simulink model "pvmodelling"  (R2022a)
settings: Solver=FixedStepAuto  StartTime=0.0  StopTime=0.33  FixedStep=0.01  MaxStep=1e-5  MinStep=1e-6  RelTol=1e-6  AbsTol=1e-6  EnableMultiTasking=on
values from neighbouring files (symbols this model uses):
  a1 = x(i,4)    [comp3.m]
  a2 = x(i,5)    [comp3.m]
  I01 = x(i,2)    [comp3.m]    (also in modified_two_diode_model2.m = (B/rp)*(rp+rs))
  I02 = x(i,3)    [comp3.m]    (also in modified_two_diode_model2.m = (E/rp)*(rp+rs))
  Iph = x(i,1)    [comp3.m]    (also in modified_two_diode_model2.m = (A/rp)*(rp+rs))
  Rp = x(i,7)    [comp3.m]
  Rs = x(i,6)    [comp3.m]
  Vt = (K11*(T)*Ns)/Q    (= 0.0828298974046)    [input2.m]
undefined symbols (not defined in the file or in its folder): sigbuilder_block
settings Model: Creator=SREEKANTHA  LastModifiedBy=abdul
settings SolverCC: AutoScaleAbsTol=off  InitialStep=1e-6  AlgebraicLoopSolver=TrustRegion
settings DataIOCC: ReturnWorkspaceOutputs=off
settings OptimizationCC: LifeSpan=inf
settings DebuggingCC: UnconnectedInputMsg=warning  UnconnectedOutputMsg=warning  UnconnectedLineMsg=warning  SFUnexpectedBacktrackingDiag=warning  SFNoUnconditionalDefaultTransitionDiag=warning  SFMachineParentedDataDiag=warning  ArithmeticOperatorsInVariantConditions=warning
settings SFSimCC: SimUseLocalCustomCode=off  CustomCodeUndefinedFunction=UseInterfaceOnly
settings RTWCC: RTWUseLocalCustomCode=off
settings CodeAppCC: StateflowObjectComments=on
settings GRTTargetCC: TargetLangStandard=C89/C90 (ANSI)
settings ConfigComp: CovMetricSettings=dw  CovSaveCumulativeToWorkspaceVar=on  CovSaveSingleToWorkspaceVar=on  CovExternalEMLEnable=off
settings SimscapeCC: SimscapeNormalizeSystem=off

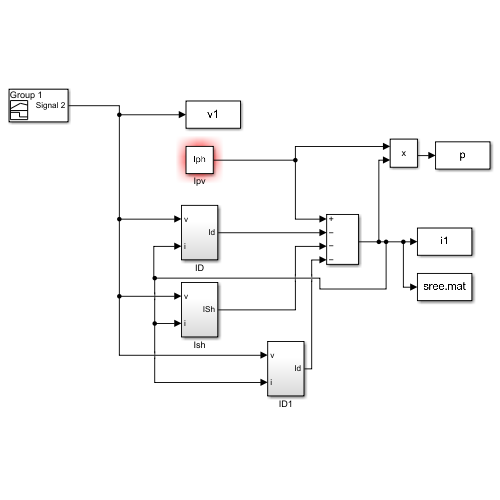
[thumbnail: Simulink's stored preview of the top-level diagram]
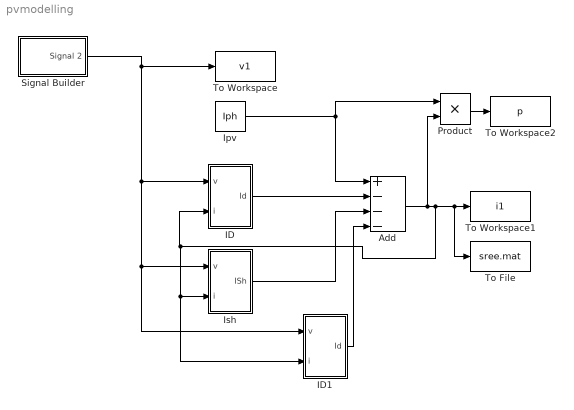
== system pvmodelling ==
  Add : Sum  Inputs=+---
  ID : Subsystem
  ID1 : Subsystem
  Ipv : Constant  Value=Iph
  Ish : Subsystem
  Product : Product
  Signal Builder : Subsystem  Tag=STV Subsys  LoadFcn=sigbuilder_block('load');  StartFcn=sigbuilder_block('start');  StopFcn=sigbuilder_block('stop');  ClipboardFcn=sigbuilder_block('clipboard');  mask(Sigbuilder block){tuvar=[0:10]}
      mask help: Simulink:masks:SigbuilderBlock_MD
      mask init:
      | if ~strcmp(get_param(bdroot(gcbh),'SimulationStatus'),'stopped') tuvar = sigbuilder_block('maskInit'); end
      settings: CopyFcn=sigbuilder_block('copy');  DeleteFcn=sigbuilder_block('delete');  ModelCloseFcn=sigbuilder_block('modelClose');  PreSaveFcn=sigbuilder_block('preSave');  PauseFcn=sigbuilder_block('pause');  ContinueFcn=sigbuilder_block('continue');  NameChangeFcn=sigbuilder_block('namechange');  OpenFcn=sigbuilder_block('open',[0 36 1152 555.6 ]);  CloseFcn=sigbuilder_block('close');
      mask Display: plot(0, 0, 100, 100,[2, 2, 32, 32, 2], [68, 8, 8, 68, 68],[32, 2], [38, 38], [32, 19, 2],[53, 60, 44], [32, 17, 17, 2],[16, 16, 31, 31]);txt = getActiveGroup(gcbh);text(2, 100, txt,'verticalAlignment', 'top');
  To File : ToFile  Filename=sree.mat  MatrixName=ii
  To Workspace : ToWorkspace  VariableName=v1  SampleTime=-1
  To Workspace1 : ToWorkspace  VariableName=i1  SampleTime=-1
  To Workspace2 : ToWorkspace  VariableName=p  SampleTime=-1
  wires:
  Ipv/1 -> Product/1, Add/1
  ID/1(Id) -> Add/2
  Ish/1(ISh) -> Add/3
  Add/1 -> Product/2, To Workspace1/1, To File/1, ID1/2(i), Ish/2(i), ID/2(i)
  Product/1 -> To Workspace2/1
  ID1/1(Id) -> Add/4
  Signal Builder/1(Signal 2) -> ID1/1(v), Ish/1(v), ID/1(v), To Workspace/1

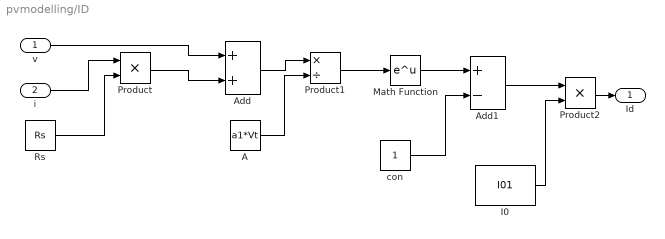
== system pvmodelling/ID ==
  v : Inport
  i : Inport  Port=2
  A : Constant  Value=a1*Vt
  Add : Sum
  Add1 : Sum  Inputs=+-
  I0 : Constant  Value=I01
  Math Function : Math  SignedPower=on
  Product : Product
  Product1 : Product  Inputs=*/
  Product2 : Product
  Rs : Constant  Value=Rs
  con : Constant
  Id : Outport
  wires:
  con/1 -> Add1/2
  Add1/1 -> Product2/1
  Product1/1 -> Math Function/1
  Product/1 -> Add/2
  I0/1 -> Product2/2
  Math Function/1 -> Add1/1
  Product2/1 -> Id/1
  v/1 -> Add/1
  Rs/1 -> Product/2
  A/1 -> Product1/2
  Add/1 -> Product1/1
  i/1 -> Product/1

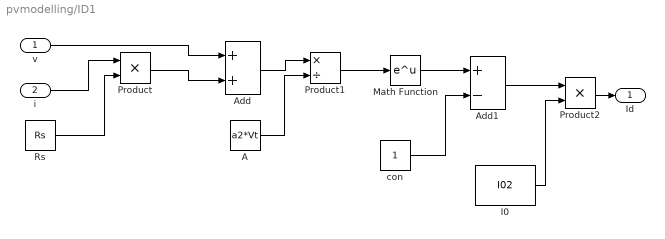
== system pvmodelling/ID1 ==
  v : Inport
  i : Inport  Port=2
  A : Constant  Value=a2*Vt
  Add : Sum
  Add1 : Sum  Inputs=+-
  I0 : Constant  Value=I02
  Math Function : Math  SignedPower=on
  Product : Product
  Product1 : Product  Inputs=*/
  Product2 : Product
  Rs : Constant  Value=Rs
  con : Constant
  Id : Outport
  wires:
  con/1 -> Add1/2
  Add1/1 -> Product2/1
  Product1/1 -> Math Function/1
  Product/1 -> Add/2
  I0/1 -> Product2/2
  Math Function/1 -> Add1/1
  Product2/1 -> Id/1
  v/1 -> Add/1
  Rs/1 -> Product/2
  A/1 -> Product1/2
  Add/1 -> Product1/1
  i/1 -> Product/1

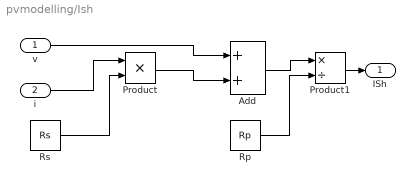
== system pvmodelling/Ish ==
  v : Inport
  i : Inport  Port=2
  Add : Sum
  Product : Product
  Product1 : Product  Inputs=*/
  Rp : Constant  Value=Rp
  Rs : Constant  Value=Rs
  ISh : Outport
  wires:
  Product1/1 -> ISh/1
  Rs/1 -> Product/2
  Rp/1 -> Product1/2
  Product/1 -> Add/2
  v/1 -> Add/1
  Add/1 -> Product1/1
  i/1 -> Product/1

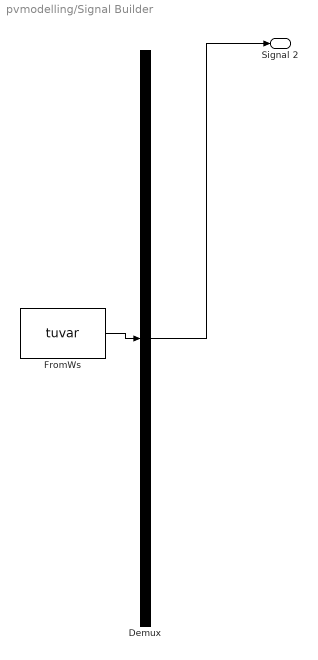
== system pvmodelling/Signal Builder ==
  Demux : Demux  Tag=STV Demux  Outputs=1
      settings: DisplayOption=none
  FromWs : FromWorkspace  Tag=STV FromWs  VariableName=tuvar
      SigBuilderData=|
      | common.afterFinalStr = 'Extrapolate'
      | common.sampleTime = 0
      | dataSet.timeRange = [0 0.33]
      | dataSet.name = 'Group 1'
      | sbobj.Groups.Name = 'Group 1'
      | sbobj.Groups.Signals.Name = 'Signal 2'
      | sbobj.Groups.Signals.XData = [0 0.01 0.02 0.03 0.04 0.05 0.06 0.07 0.08 0.09 0.1 0.11 0.12 0.13 0.14 0.15 0.16 0.17 0.18 0.19 0.2 0.21 0.22 0.23 0.24 0.25 0.26 0.27 0.28 0.29 0.3 0.31 0.32 0.33]
      | sbobj.Groups.Signals.YData = [0 12.2 14.7 15.7 16.2 17 17.3 17.7 18 18.3 18.5 18.8 19 19.2 19.4 19.5 19.7 19.8 20 20.1 20.3 20.4 20.5 20.6 20.7 20.8 20.9 21 21.1 21.2 21.3 21.4 21.5 21.6]
      | sbobj.Groups.TimeRange = [0 0.33]
  Signal 2 : Outport  Tag=STV Outport
  wires:
  FromWs/1 -> Demux/1
  Demux/1 -> Signal 2/1
